simulink model "Wk1_Q1"  (R2022b)
settings: Solver=VariableStepAuto  StartTime=0.0  StopTime=5  RelTol=1e-3
values from neighbouring files (symbols this model uses):
  g = 9.81    [Wk1_Q1_2_3_6_7_8.m]
  l = 1    [Wk1_Q1_2_3_6_7_8.m]
  m = 1    [Wk1_Q1_2_3_6_7_8.m]
  tau = 0    [Wk1_Q1_2_3_6_7_8.m]
  Theta = pi/2    (= 1.57079632679)    [Wk1_Q1_2_3_6_7_8.m]
  Thetadot = 0    [Wk1_Q1_2_3_6_7_8.m]
settings Model: Creator=zd012  LastModifiedBy=zd012
settings DebuggingCC: UnconnectedInputMsg=warning  UnconnectedOutputMsg=warning  UnconnectedLineMsg=warning
settings ModelReferenceCC: EnableRefExpFcnMdlSchedulingChecks=on
settings RTWCC: DLArmComputeVersion=19.05

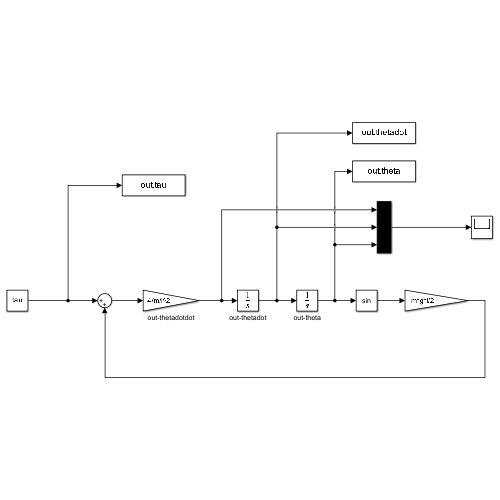
[thumbnail: Simulink's stored preview of the top-level diagram]
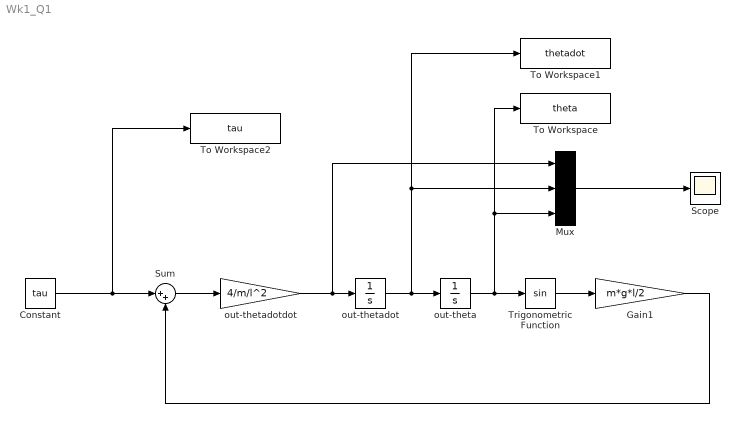
== system Wk1_Q1 ==
  Constant : Constant  Value=tau
  Gain1 : Gain  Gain=m*g*l/2
  Mux : Mux  Inputs=3
  Scope : Scope
  Sum : Sum  Inputs=|++
  To Workspace : ToWorkspace  VariableName=theta  SampleTime=-1
      settings: Save2DSignal=2-D array (concatenate along first dimension)
  To Workspace1 : ToWorkspace  VariableName=thetadot  SampleTime=-1
      settings: Save2DSignal=2-D array (concatenate along first dimension)
  To Workspace2 : ToWorkspace  VariableName=tau  SampleTime=-1
      settings: Save2DSignal=2-D array (concatenate along first dimension)
  Trigonometric Function : Trigonometry
  out-theta : Integrator  InitialCondition=Theta
  out-thetadot : Integrator  InitialCondition=Thetadot
  out-thetadotdot : Gain  Gain=4/m/l^2
  wires:
  Constant/1 -> To Workspace2/1, Sum/1
  out-thetadot/1 -> To Workspace1/1, Mux/2, out-theta/1
  Sum/1 -> out-thetadotdot/1
  out-thetadotdot/1 -> Mux/1, out-thetadot/1
  out-theta/1 -> To Workspace/1, Mux/3, Trigonometric Function/1
  Trigonometric Function/1 -> Gain1/1
  Gain1/1 -> Sum/2
  Mux/1 -> Scope/1
